simulink model "Joystick_Demo"  (R2018a)
settings: Solver=FixedStepAuto  StartTime=0.0  StopTime=inf  FixedStep=.25  RelTol=1e-3  EnableMultiTasking=on
libraries: arduinolib x10, simulink x5
settings Model: SimulationMode=external  ExtModeTrigDuration=2  Creator=jonathancoulter  LastModifiedBy=jonathancoulter
settings SolverCC: AutoInsertRateTranBlk=on
settings OptimizationCC: DefaultParameterBehavior=Inlined  UseFloatMulNetSlope=on  InlineInvariantSignals=on  PassReuseOutputArgsThreshold=0  EfficientFloat2IntCast=on  MaxStackSize=64
settings DebuggingCC: ParameterTunabilityLossMsg=error
settings HardwareCC: ProdBitPerInt=16  ProdBitPerPointer=16  ProdBitPerSizeT=16  ProdBitPerPtrDiffT=16  ProdLargestAtomicFloat=None  ProdWordSize=8  ProdHWDeviceType=Atmel->AVR  UseEmbeddedCoderFeatures=off
settings SFSimCC: MATLABDynamicMemAlloc=off
settings RTWCC: SystemTargetFile=ert.tlc  HardwareBoard=Arduino Mega 2560  TLCOptions=-aInlineSetEventsForThisBaseRateFcn=TLC_FALSE -aSuppressMultiTaskScheduler=TLC_FALSE -aRateBasedStepFcn=1  TemplateMakefile=ert_default_tmf  Toolchain=Arduino AVR  BuildConfiguration=Faster Runs  CheckMdlBeforeBuild=Warning
settings CodeAppCC: ForceParamTrailComments=on  OperatorAnnotations=on  StateflowObjectComments=on  MATLABSourceComments=on
settings ERTTargetCC: ERTCustomFileBanners=off  SupportNonFinite=off  SupportContinuousTime=on  SupportNonInlinedSFcns=on  RemoveResetFunc=off  SupportVariableSizeSignals=on  ModelStepFunctionPrototypeControlCompliant=off  InlinedParameterPlacement=NonHierarchical

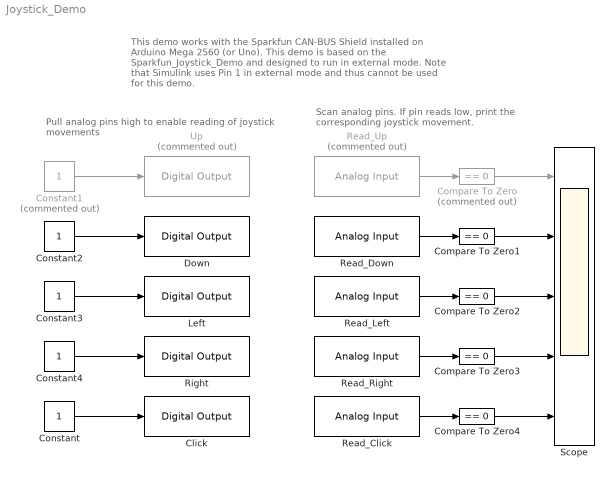
== system Joystick_Demo ==
  note: Pull analog pins high to enable reading of joystick movements
  note: This demo works with the Sparkfun CAN-BUS Shield installed on Arduino Mega 2560 (or Uno).
      | This demo is based on the Sparkfun_Joystick_Demo and designed to run in external mode.
      | Note that Simulink uses Pin 1 in external mode and thus cannot be used for this demo.
  note: Scan analog pins. If pin reads low, print the corresponding joystick movement.
  Click : arduinolib/Digital Output  pinNumber=4  blockPlatform=arduino
  Compare To Zero : simulink/Logic and Bit Operations/Compare To Zero  Commented=on  relop===  OutDataTypeStr=boolean
  Compare To Zero{1..4} (4 alike) : simulink/Logic and Bit Operations/Compare To Zero  relop===  OutDataTypeStr=boolean
  Constant{,2..4} (4 alike) : Constant  OutDataTypeStr=uint8
  Constant1 : Constant  Commented=on  OutDataTypeStr=uint8
  Down : arduinolib/Digital Output  pinNumber=3  blockPlatform=arduino
  Left : arduinolib/Digital Output  pinNumber=2  blockPlatform=arduino
  Read_Click : arduinolib/Analog Input  pinNumber=4  ReadResultsOnly=off  ConversionTriggerSource=Software  ExternalTriggerType=uint32(0)  OutputDataType=uint16  EnableConversionCompleteNotify=off  EnableOuputStatus=off  SampleTime=-1  blockPlatform=arduino
  Read_Down : arduinolib/Analog Input  pinNumber=3  ReadResultsOnly=off  ConversionTriggerSource=Software  ExternalTriggerType=uint32(0)  OutputDataType=uint16  EnableConversionCompleteNotify=off  EnableOuputStatus=off  SampleTime=-1  blockPlatform=arduino
  Read_Left : arduinolib/Analog Input  pinNumber=2  ReadResultsOnly=off  ConversionTriggerSource=Software  ExternalTriggerType=uint32(0)  OutputDataType=uint16  EnableConversionCompleteNotify=off  EnableOuputStatus=off  SampleTime=-1  blockPlatform=arduino
  Read_Right : arduinolib/Analog Input  pinNumber=5  ReadResultsOnly=off  ConversionTriggerSource=Software  ExternalTriggerType=uint32(0)  OutputDataType=uint16  EnableConversionCompleteNotify=off  EnableOuputStatus=off  SampleTime=-1  blockPlatform=arduino
  Read_Up : arduinolib/Analog Input  Commented=on  pinNumber=1  ReadResultsOnly=off  ConversionTriggerSource=Software  ExternalTriggerType=uint32(0)  OutputDataType=uint16  EnableConversionCompleteNotify=off  EnableOuputStatus=off  SampleTime=-1  blockPlatform=arduino
  Right : arduinolib/Digital Output  pinNumber=5  blockPlatform=arduino
  Scope : Scope  NumInputPorts=5
  Up : arduinolib/Digital Output  Commented=on  pinNumber=1  blockPlatform=arduino
  wires:
  Constant/1 -> Click/1
  Constant1/1 -> Up/1
  Constant2/1 -> Down/1
  Constant3/1 -> Left/1
  Constant4/1 -> Right/1
  Read_Up/1 -> Compare To Zero/1
  Read_Down/1 -> Compare To Zero1/1
  Read_Left/1 -> Compare To Zero2/1
  Read_Right/1 -> Compare To Zero3/1
  Read_Click/1 -> Compare To Zero4/1
  Compare To Zero/1 -> Scope/1
  Compare To Zero1/1 -> Scope/2
  Compare To Zero2/1 -> Scope/3
  Compare To Zero3/1 -> Scope/4
  Compare To Zero4/1 -> Scope/5
